simulink model "ASM_Traffic_V2X_Complete_Model_2"  (R2019a)
settings: Solver=ode1  StartTime=SIM.tstart.v  StopTime=Inf  FixedStep=SIM.StepSize.v  RelTol=1e-3
PostLoadFcn:
  | if any(exist('dsrtsu_mdlpostloadfcn', 'file') ~= 0), dsrtsu_mdlpostloadfcn('Execute', bdroot); end
  | try, asm_mdl_postloadfcn(bdroot, 'UpdateModel', 2200); catch, disp(lasterr); end,
undefined symbols (not defined in the file): _SensorPnts_1, _SensorPnts_13, _SensorPnts_17, _SensorPnts_21, _SensorPnts_25, _SensorPnts_29, _SensorPnts_33, _SensorPnts_37, _SensorPnts_41, _SensorPnts_45, _SensorPnts_49, _SensorPnts_5, _SensorPnts_53, _SensorPnts_57, _SensorPnts_9, _to_, CPT, G5A, ITS, MDL, rad, s_to_rpm, SIM
libraries: simulink x169, ASM_VehicleDynamics_lib x126, ASM_Traffic_lib x83, ASM_Utils_lib x49, mdbs x45, ASM_Environment_lib x17, dspindex x12, dsaV2xLibraryAux x10, dsmpblib x6, dsaV2xAsn1Library x4, dsaV2xLibrary x4, ASM_BrakeHydraulics_lib x4
(part 16 of 36)

== system ASM_Traffic_V2X_Complete_Model_2/MDLUserInterface/MotionDeskInterface/Fellow_VehicleLights/Fellow9 ==
  SW_Signals_UserInterface : Inport
  v_fellow[m|s] : Inport  Port=2
  TurnLights[0|1|2|3] : Inport  Port=3
  Acceleration[m|s2] : simulink/Discrete/Discrete Derivative  gainval=1.0  ICPrevScaledInput=0.0  OutMin=[]  OutMax=[]  OutDataType=fixdt(1, 16)  OutScaling=2^-10  DoSatur=off
  Bus Selector : BusSelector  OutputSignals=SW_ManualControl_Lights[1Scheduler|2Manual],SW_BrakeLight[0Off|1On],SW_TurnLights[0Off|1Left|2Right|3Both]
  Compare_Both : simulink/Logic and Bit Operations/Compare To Constant  relop===  const=3  OutDataTypeStr=boolean
  Compare_Brakelight : simulink/Logic and Bit Operations/Compare To Constant  relop=<  const=-0.2  OutDataTypeStr=boolean
  Compare_Turnlight_L : simulink/Logic and Bit Operations/Compare To Constant  relop===  const=1  OutDataTypeStr=boolean
  Compare_Turnlight_R : simulink/Logic and Bit Operations/Compare To Constant  relop===  const=2  OutDataTypeStr=boolean
  Data Type Conversion1 : DataTypeConversion  OutDataTypeStr=boolean
  Data Type Conversion2 : DataTypeConversion  OutDataTypeStr=uint32
  Data Type Conversion3 : DataTypeConversion  OutDataTypeStr=uint32
  Data Type Conversion4 : DataTypeConversion  OutDataTypeStr=uint32
  Logical Operator : Logic  Operator=OR  AllPortsSameDT=off  OutDataTypeStr=boolean
  Logical Operator1 : Logic  Operator=OR  AllPortsSameDT=off  OutDataTypeStr=boolean
  Multiport Switch : MultiPortSwitch  Inputs=2
  Multiport Switch4 : MultiPortSwitch  Inputs=2
  Mux16 : Mux  Inputs=3
  FellowLights : Outport
  wires:
  Data Type Conversion4/1 -> Multiport Switch4/2
  Data Type Conversion2/1 -> Multiport Switch4/3
  Data Type Conversion1/1 -> Multiport Switch/3
  Data Type Conversion3/1 -> Multiport Switch4/1, Multiport Switch/1
  SW_Signals_UserInterface/1 -> Bus Selector/1
  Acceleration[m|s2]/1 -> Compare_Brakelight/1
  Mux16/1 -> FellowLights/1
  TurnLights[0|1|2|3]/1 -> Data Type Conversion4/1
  v_fellow[m|s]/1 -> Acceleration[m|s2]/1
  Bus Selector/3 -> Data Type Conversion2/1  "<SW_TurnLights[0Off|1Left|2Right|3Both]>"
  Multiport Switch4/1 -> Compare_Both/1, Compare_Turnlight_R/1, Compare_Turnlight_L/1
  Logical Operator1/1 -> Mux16/3
  Logical Operator/1 -> Mux16/2
  Compare_Both/1 -> Logical Operator/2, Logical Operator1/2
  Compare_Turnlight_R/1 -> Logical Operator1/1
  Compare_Turnlight_L/1 -> Logical Operator/1
  Multiport Switch/1 -> Mux16/1
  Bus Selector/2 -> Data Type Conversion1/1  "<SW_BrakeLight[0Off|1On]>"
  Compare_Brakelight/1 -> Multiport Switch/2
  Bus Selector/1 -> Data Type Conversion3/1  "<SW_ManualControl_Lights[1Scheduler|2Manual]>"

== system ASM_Traffic_V2X_Complete_Model_2/MDLUserInterface/MotionDeskInterface/MOTION_DESK_INTERFACE/CalcLDWState ==
  NetworkItemType[] : Inport
  Dist_L[m] : Inport  Port=2
  Dist_R[m] : Inport  Port=3
  Compare To Constant : simulink/Logic and Bit Operations/Compare To Constant  relop===  const=3  OutDataTypeStr=boolean
  EvaluateDistance_L : If  IfExpression=u1 <= 0.01  ElseIfExpressions=(u1>0.01 & u1<=0.2)
  EvaluateDistance_R : If  IfExpression=u1 <= 0.01  ElseIfExpressions=(u1>0.01 & u1<=0.2)
  Junction : Constant  Value=0
  LeavingLane_L : Subsystem  TreatAsAtomicUnit=on
  LeavingLane_R : Subsystem  TreatAsAtomicUnit=on
  Merge : Merge  Inputs=3
  Merge1 : Merge  Inputs=3
  OK_L : Subsystem  TreatAsAtomicUnit=on
  OK_R : Subsystem  TreatAsAtomicUnit=on
  OutOfLane_L : Subsystem  TreatAsAtomicUnit=on
  OutOfLane_R : Subsystem  TreatAsAtomicUnit=on
  Switch : Switch  Criteria=u2 > Threshold
  Switch1 : Switch  Criteria=u2 > Threshold
  LDWState_L[] : Outport
  LDWState_R[] : Outport  Port=2
  wires:
  Merge1/1 -> Switch1/3
  Dist_R[m]/1 -> EvaluateDistance_R/1
  EvaluateDistance_R/1 -> OutOfLane_R/Action
  EvaluateDistance_R/2 -> LeavingLane_R/Action
  EvaluateDistance_R/3 -> OK_R/Action
  OutOfLane_R/1(Out1) -> Merge1/1
  LeavingLane_R/1(Out1) -> Merge1/2
  OK_R/1(Out1) -> Merge1/3
  Merge/1 -> Switch/3
  OK_L/1(Out1) -> Merge/3
  LeavingLane_L/1(Out1) -> Merge/2
  OutOfLane_L/1(Out1) -> Merge/1
  EvaluateDistance_L/3 -> OK_L/Action
  EvaluateDistance_L/2 -> LeavingLane_L/Action
  EvaluateDistance_L/1 -> OutOfLane_L/Action
  Dist_L[m]/1 -> EvaluateDistance_L/1
  Switch1/1 -> LDWState_R[]/1
  Junction/1 -> Switch/1, Switch1/1
  Switch/1 -> LDWState_L[]/1
  Compare To Constant/1 -> Switch/2, Switch1/2
  NetworkItemType[]/1 -> Compare To Constant/1

== system ASM_Traffic_V2X_Complete_Model_2/MDLUserInterface/MotionDeskInterface/MOTION_DESK_INTERFACE/Chassis ==
  Transform_In : Inport
  Pos_Vehicle_CoorSys_E[x;y;z][m] : Inport  Port=2
  Angle_Vehicle_CoorSys_E[x;y;z][deg] : Inport  Port=3
  MD_Object : mdbs/MD_Object  strObjId=0  strObjName=chassis  strBlockType=OBJ  bGUIEventOK=0
      settings: SourceProductName=dSPACE MotionDesk Blockset
  Selector : Selector  InputPortWidth=3  IndexOptions=Index vector (dialog)  Indices=[3 2 1]  OutputSizes=1
  Transform_Out : Outport
  wires:
  Selector/1 -> MD_Object/3
  Transform_In/1 -> MD_Object/1
  MD_Object/1 -> Transform_Out/1
  Pos_Vehicle_CoorSys_E[x;y;z][m]/1 -> MD_Object/2
  Angle_Vehicle_CoorSys_E[x;y;z][deg]/1 -> Selector/1

== system ASM_Traffic_V2X_Complete_Model_2/MDLUserInterface/MotionDeskInterface/MOTION_DESK_INTERFACE/Coding ==
  In1 : Inport
  Bitwise Operator3 : simulink/Logic and Bit Operations/Bitwise Operator  logicop=OR  UseBitMask=off  NumInputPorts=3  BitMask=bin2dec('11011001')  BitMaskRealWorld=Stored Integer
  Data Type Conversion : DataTypeConversion  OutDataTypeStr=uint32
  Data Type Conversion1 : DataTypeConversion  OutDataTypeStr=uint32
  Demux : Demux  Outputs=3
  Gain : Gain  Gain=15  ParamDataTypeStr=uint32  OutDataTypeStr=uint32
  Gain1 : Gain  Gain=15  ParamDataTypeStr=uint32  OutDataTypeStr=uint32
  Gain2 : Gain  Gain=15  ParamDataTypeStr=uint32  OutDataTypeStr=uint32
  Shift Arithmetic : ArithShift  BitShiftNumber=4  BitShiftDirection=Left
  Shift Arithmetic1 : ArithShift  BitShiftNumber=8  BitShiftDirection=Left
  SwitchDelay : Subsystem
  Out1 : Outport
  wires:
  Data Type Conversion1/1 -> Out1/1
  Bitwise Operator3/1 -> Data Type Conversion1/1
  Demux/1 -> Gain/1
  Data Type Conversion/1 -> Demux/1
  Shift Arithmetic1/1 -> Bitwise Operator3/3
  Shift Arithmetic/1 -> Bitwise Operator3/2
  Gain2/1 -> Shift Arithmetic1/1
  Gain1/1 -> Shift Arithmetic/1
  Gain/1 -> Bitwise Operator3/1
  In1/1 -> Data Type Conversion/1
  Demux/2 -> SwitchDelay/1(Turnlight_L)
  Demux/3 -> SwitchDelay/2(Turnlight_R)
  SwitchDelay/1(Turnlight_L_out) -> Gain1/1
  SwitchDelay/2(Turnlight_R_out) -> Gain2/1

== system ASM_Traffic_V2X_Complete_Model_2/MDLUserInterface/MotionDeskInterface/MOTION_DESK_INTERFACE/Coding_Fellows ==
  In1 : Inport
  Coding1 : Subsystem
  Coding10 : Subsystem
  Coding11 : Subsystem
  Coding12 : Subsystem
  Coding13 : Subsystem
  Coding14 : Subsystem
  Coding15 : Subsystem
  Coding2 : Subsystem
  Coding3 : Subsystem
  Coding4 : Subsystem
  Coding5 : Subsystem
  Coding6 : Subsystem
  Coding7 : Subsystem
  Coding8 : Subsystem
  Coding9 : Subsystem
  Demux : Demux  Outputs=15
  Mux : Mux  Inputs=15
  Out1 : Outport
  wires:
  In1/1 -> Demux/1
  Coding1/1(Out1) -> Mux/1
  Mux/1 -> Out1/1
  Coding2/1(Out1) -> Mux/2
  Coding3/1(Out1) -> Mux/3
  Coding4/1(Out1) -> Mux/4
  Coding5/1(Out1) -> Mux/5
  Coding6/1(Out1) -> Mux/6
  Coding7/1(Out1) -> Mux/7
  Coding8/1(Out1) -> Mux/8
  Coding9/1(Out1) -> Mux/9
  Coding10/1(Out1) -> Mux/10
  Coding11/1(Out1) -> Mux/11
  Coding12/1(Out1) -> Mux/12
  Coding13/1(Out1) -> Mux/13
  Coding14/1(Out1) -> Mux/14
  Coding15/1(Out1) -> Mux/15
  Demux/1 -> Coding1/1(In1)
  Demux/2 -> Coding2/1(In1)
  Demux/3 -> Coding3/1(In1)
  Demux/4 -> Coding4/1(In1)
  Demux/5 -> Coding5/1(In1)
  Demux/6 -> Coding6/1(In1)
  Demux/7 -> Coding7/1(In1)
  Demux/8 -> Coding8/1(In1)
  Demux/9 -> Coding9/1(In1)
  Demux/10 -> Coding10/1(In1)
  Demux/11 -> Coding11/1(In1)
  Demux/12 -> Coding12/1(In1)
  Demux/13 -> Coding13/1(In1)
  Demux/14 -> Coding14/1(In1)
  Demux/15 -> Coding15/1(In1)

== system ASM_Traffic_V2X_Complete_Model_2/MDLUserInterface/MotionDeskInterface/MOTION_DESK_INTERFACE/FrontAxle ==
  Transform_In : Inport
  Pos_Wheel_L[x;y;z][m] : Inport  Port=2
  AngleWheel_L[z;x][deg] : Inport  Port=3
  AngleWheel_L[y][deg] : Inport  Port=4
  r_Dyn_Tire_L[m] : Inport  Port=5
  F_Tire_L_CoorSys_V[x;y;z][N] : Inport  Port=6
  Pos_Wheel_R[x;y;z][m] : Inport  Port=7
  AngleWheel_R[z;x][deg] : Inport  Port=8
  AngleWheel_R[y][deg] : Inport  Port=9
  r_Dyn_Tire_R[m] : Inport  Port=10
  F_Tire_R_CoorSys_V[x;y;z][N] : Inport  Port=11
  Constant1 : Constant
  Constant2 : Constant  Value=0
  Constant8 : Constant  Value=0.36
  Demux2 : Demux  Outputs=3
  Demux4 : Demux  Outputs=3
  Divide : Product  Inputs=*/
  Divide1 : Product  Inputs=*/
  MD_Object1 : mdbs/MD_Object  strObjId=1  strObjName=wheel_FL  strBlockType=OBJ  bGUIEventOK=0
      settings: SourceProductName=dSPACE MotionDesk Blockset
  MD_Object2 : mdbs/MD_Object  strObjId=3  strObjName=_TireFrcs_F_LR  strBlockType=OBJ  bGUIEventOK=0
      settings: SourceProductName=dSPACE MotionDesk Blockset
  MD_Object5 : mdbs/MD_Object  strObjId=2  strObjName=wheel_FR  strBlockType=OBJ  bGUIEventOK=0
      settings: SourceProductName=dSPACE MotionDesk Blockset
  Mux{,1,4,8} (4 alike) : Mux  Inputs=3
  Mux2 : Mux  Inputs=8
  Mux3 : Mux  Inputs=2
  Mux5 : Mux  Inputs=2
  Pos_z_Offset_Arrow[m] : Constant  Value=0.1
  Product1 : Product  SaturateOnIntegerOverflow=on  OutDataTypeStr=Inherit: Same as first input
  Product2 : Product  SaturateOnIntegerOverflow=on  OutDataTypeStr=Inherit: Same as first input
  Reshape : Reshape  OutputDimensionality=Customize  OutputDimensions=[4,4]
  ScalingFaktor_F_Tire[] : Constant  Value=0.001
  Sign : Gain  Gain=-1
  Sum : Sum  Inputs=+-+  SaturateOnIntegerOverflow=on  InputSameDT=on  OutDataTypeStr=Inherit: Same as first input
  Sum1 : Sum  Inputs=+-+  SaturateOnIntegerOverflow=on  InputSameDT=on  OutDataTypeStr=Inherit: Same as first input
  Terminator1 : Terminator
  Terminator2 : Terminator
  Terminator5 : Terminator
  wires:
  AngleWheel_R[z;x][deg]/1 -> Mux5/1
  Sign/1 -> Mux3/1
  Mux5/1 -> MD_Object5/3
  Mux3/1 -> MD_Object1/3
  Reshape/1 -> MD_Object2/1
  Mux2/1 -> Reshape/1
  Constant2/1 -> Mux2/2, Mux2/4, Mux2/6, Mux2/8
  Product1/1 -> Mux2/7
  Mux1/1 -> Mux2/5
  Product2/1 -> Mux2/3
  Mux/1 -> Mux2/1
  AngleWheel_R[y][deg]/1 -> Mux5/2
  Transform_In/1 -> MD_Object1/1, MD_Object5/1
  r_Dyn_Tire_R[m]/1 -> Divide1/1, Sum1/2
  Constant1/1 -> Mux4/2, Mux8/2
  Mux8/1 -> MD_Object5/4
  Constant8/1 -> Divide/2, Divide1/2
  Divide1/1 -> Mux8/3, Mux8/1
  Pos_z_Offset_Arrow[m]/1 -> Sum1/3, Sum/3
  Sum1/1 -> Mux1/3
  Demux4/3 -> Sum1/1
  Demux4/2 -> Mux1/2
  Demux4/1 -> Mux1/1
  Pos_Wheel_R[x;y;z][m]/1 -> Demux4/1, MD_Object5/2
  ScalingFaktor_F_Tire[]/1 -> Product1/2, Product2/2
  F_Tire_R_CoorSys_V[x;y;z][N]/1 -> Product1/1
  MD_Object5/1 -> Terminator5/1
  MD_Object2/1 -> Terminator2/1
  MD_Object1/1 -> Terminator1/1
  F_Tire_L_CoorSys_V[x;y;z][N]/1 -> Product2/1
  Pos_Wheel_L[x;y;z][m]/1 -> MD_Object1/2, Demux2/1
  Demux2/1 -> Mux/1
  Demux2/2 -> Mux/2
  Demux2/3 -> Sum/1
  Sum/1 -> Mux/3
  Divide/1 -> Mux4/1, Mux4/3
  Mux4/1 -> MD_Object1/4
  r_Dyn_Tire_L[m]/1 -> Sum/2, Divide/1
  AngleWheel_L[z;x][deg]/1 -> Sign/1
  AngleWheel_L[y][deg]/1 -> Mux3/2

== system ASM_Traffic_V2X_Complete_Model_2/MDLUserInterface/MotionDeskInterface/MOTION_DESK_INTERFACE/LaneSensor1_L ==
  Transform_In : Inport
  Pos_Sensor[x;y;z][m] : Inport  Port=2
  Angle_Yaw[deg] : Inport  Port=3
  Scaling : Inport  Port=4
  Constant1 : Constant  Value=0
  Constant4 : Constant  Value=0
  MD_Object : mdbs/MD_Object  strObjId=38  strObjName=LaneSensor_Left  strBlockType=OBJ  bGUIEventOK=0
      settings: SourceProductName=dSPACE MotionDesk Blockset
  Mux : Mux  Inputs=3
  Mux1 : Mux  Inputs=3
  Terminator1 : Terminator
  wires:
  MD_Object/1 -> Terminator1/1
  Pos_Sensor[x;y;z][m]/1 -> MD_Object/2
  Transform_In/1 -> MD_Object/1
  Mux1/1 -> MD_Object/3
  Constant4/1 -> Mux1/3
  Constant1/1 -> Mux1/2
  Angle_Yaw[deg]/1 -> Mux1/1
  Mux/1 -> MD_Object/4
  Scaling/1 -> Mux/3, Mux/1, Mux/2

== system ASM_Traffic_V2X_Complete_Model_2/MDLUserInterface/MotionDeskInterface/MOTION_DESK_INTERFACE/LaneSensor1_R ==
  Transform_In : Inport
  Pos_Sensor[x;y;z][m] : Inport  Port=2
  Angle_Yaw[deg] : Inport  Port=3
  Scaling : Inport  Port=4
  Constant1 : Constant  Value=0
  Constant4 : Constant  Value=0
  MD_Object : mdbs/MD_Object  strObjId=39  strObjName=LaneSensor_Right  strBlockType=OBJ  bGUIEventOK=0
      settings: SourceProductName=dSPACE MotionDesk Blockset
  Mux : Mux  Inputs=3
  Mux1 : Mux  Inputs=3
  Terminator1 : Terminator
  wires:
  Constant4/1 -> Mux1/3
  Mux1/1 -> MD_Object/3
  Transform_In/1 -> MD_Object/1
  Pos_Sensor[x;y;z][m]/1 -> MD_Object/2
  MD_Object/1 -> Terminator1/1
  Constant1/1 -> Mux1/2
  Angle_Yaw[deg]/1 -> Mux1/1
  Scaling/1 -> Mux/3, Mux/1, Mux/2
  Mux/1 -> MD_Object/4

== system ASM_Traffic_V2X_Complete_Model_2/MDLUserInterface/MotionDeskInterface/MOTION_DESK_INTERFACE/RearAxle ==
  Transform_In : Inport
  Pos_Wheel_L[x;y;z][m] : Inport  Port=2
  AngleWheel_L[z;x][deg] : Inport  Port=3
  AngleWheel_L[y][deg] : Inport  Port=4
  r_Dyn_Tire_L[m] : Inport  Port=5
  F_Tire_L_CoorSys_V[x;y;z][N] : Inport  Port=6
  Pos_Wheel_R[x;y;z][m] : Inport  Port=7
  AngleWheel_R[z;x][deg] : Inport  Port=8
  AngleWheel_R[y][deg] : Inport  Port=9
  r_Dyn_Tire_R[m] : Inport  Port=10
  F_Tire_R_CoorSys_V[x;y;z][N] : Inport  Port=11
  Constant1 : Constant
  Constant2 : Constant  Value=0
  Constant8 : Constant  Value=0.36
  Demux2 : Demux  Outputs=3
  Demux4 : Demux  Outputs=3
  Divide : Product  Inputs=*/
  Divide1 : Product  Inputs=*/
  MD_Object1 : mdbs/MD_Object  strObjId=4  strObjName=wheel_RL  strBlockType=OBJ  bGUIEventOK=0
      settings: SourceProductName=dSPACE MotionDesk Blockset
  MD_Object5 : mdbs/MD_Object  strObjId=5  strObjName=wheel_RR  strBlockType=OBJ  bGUIEventOK=0
      settings: SourceProductName=dSPACE MotionDesk Blockset
  MD_Object6 : mdbs/MD_Object  strObjId=6  strObjName=_TireFrcs_R_LR  strBlockType=OBJ  bGUIEventOK=0
      settings: SourceProductName=dSPACE MotionDesk Blockset
  Mux{,1,4,8} (4 alike) : Mux  Inputs=3
  Mux2 : Mux  Inputs=8
  Mux3 : Mux  Inputs=2
  Mux5 : Mux  Inputs=2
  Pos_z_Offset_Arrow[m] : Constant  Value=0.1
  Product1 : Product  SaturateOnIntegerOverflow=on  OutDataTypeStr=Inherit: Same as first input
  Product2 : Product  SaturateOnIntegerOverflow=on  OutDataTypeStr=Inherit: Same as first input
  Reshape : Reshape  OutputDimensionality=Customize  OutputDimensions=[4,4]
  ScalingFaktor_F_Tire[] : Constant  Value=0.001
  Sign : Gain  Gain=-1
  Sum : Sum  Inputs=+-+  SaturateOnIntegerOverflow=on  InputSameDT=on  OutDataTypeStr=Inherit: Same as first input
  Sum1 : Sum  Inputs=+-+  SaturateOnIntegerOverflow=on  InputSameDT=on  OutDataTypeStr=Inherit: Same as first input
  Terminator1 : Terminator
  Terminator5 : Terminator
  Terminator6 : Terminator
  wires:
  Sign/1 -> Mux3/1
  Mux5/1 -> MD_Object5/3
  Mux3/1 -> MD_Object1/3
  Product1/1 -> Mux2/7
  Mux1/1 -> Mux2/5
  Product2/1 -> Mux2/3
  Mux/1 -> Mux2/1
  Reshape/1 -> MD_Object6/1
  Mux2/1 -> Reshape/1
  Constant2/1 -> Mux2/2, Mux2/4, Mux2/6, Mux2/8
  MD_Object5/1 -> Terminator5/1
  MD_Object6/1 -> Terminator6/1
  F_Tire_R_CoorSys_V[x;y;z][N]/1 -> Product1/1
  ScalingFaktor_F_Tire[]/1 -> Product2/2, Product1/2
  Pos_Wheel_R[x;y;z][m]/1 -> MD_Object5/2, Demux4/1
  Demux4/1 -> Mux1/1
  Demux4/2 -> Mux1/2
  Demux4/3 -> Sum1/1
  Sum1/1 -> Mux1/3
  Pos_z_Offset_Arrow[m]/1 -> Sum/3, Sum1/3
  Divide1/1 -> Mux8/1, Mux8/3
  Constant8/1 -> Divide/2, Divide1/2
  Mux8/1 -> MD_Object5/4
  Constant1/1 -> Mux4/2, Mux8/2
  r_Dyn_Tire_R[m]/1 -> Sum1/2, Divide1/1
  Transform_In/1 -> MD_Object1/1, MD_Object5/1
  AngleWheel_R[z;x][deg]/1 -> Mux5/1
  AngleWheel_R[y][deg]/1 -> Mux5/2
  MD_Object1/1 -> Terminator1/1
  F_Tire_L_CoorSys_V[x;y;z][N]/1 -> Product2/1
  Pos_Wheel_L[x;y;z][m]/1 -> Demux2/1, MD_Object1/2
  Demux2/1 -> Mux/1
  Demux2/2 -> Mux/2
  Demux2/3 -> Sum/1
  Sum/1 -> Mux/3
  Divide/1 -> Mux4/1, Mux4/3
  Mux4/1 -> MD_Object1/4
  r_Dyn_Tire_L[m]/1 -> Sum/2, Divide/1
  AngleWheel_L[z;x][deg]/1 -> Sign/1
  AngleWheel_L[y][deg]/1 -> Mux3/2

== system ASM_Traffic_V2X_Complete_Model_2/MDLUserInterface/MotionDeskInterface/MOTION_DESK_INTERFACE/SteeringWheel ==
  Transform_In : Inport
  Angle_SteeringWheel[deg] : Inport  Port=2
  Angle_inclination[deg] : Constant  Value=205
  MD_Object3 : mdbs/MD_Object  strObjId=7  strObjName=steering_wheel  strBlockType=OBJ  bGUIEventOK=0
      settings: SourceProductName=dSPACE MotionDesk Blockset
  Mux : Mux  Inputs=3
  Pos_SteeringWheel[m] : Constant  Value=[-1.3, 0.35, 0.53]
  Terminator3 : Terminator
  const : Constant  Value=0
  wires:
  Angle_SteeringWheel[deg]/1 -> Mux/3
  Pos_SteeringWheel[m]/1 -> MD_Object3/2
  Mux/1 -> MD_Object3/3
  Transform_In/1 -> MD_Object3/1
  Angle_inclination[deg]/1 -> Mux/2
  const/1 -> Mux/1
  MD_Object3/1 -> Terminator3/1

== system ASM_Traffic_V2X_Complete_Model_2/MDLUserInterface/MotionDeskInterface/MOTION_DESK_INTERFACE/Traffic_Animation ==
  Transform_In : Inport
  Pos_Fellows_MainPnt_CoorSys_E[x;y;z][m] : Inport  Port=2
  Angle_Fellows[x;y;z][deg] : Inport  Port=3
  Flag_FellowsUsed[0|1] : Inport  Port=4
  Sensors_Signals : Inport  Port=5
  Fellows_Animation : Subsystem
  Sensors_Animation : Subsystem
  wires:
  Transform_In/1 -> Sensors_Animation/1(Transform_In)
  Sensors_Signals/1 -> Sensors_Animation/2(Sensors_Signals)
  Flag_FellowsUsed[0|1]/1 -> Fellows_Animation/3(Flag_FellowsUsed[0|1])
  Pos_Fellows_MainPnt_CoorSys_E[x;y;z][m]/1 -> Fellows_Animation/1(Pos_Fellows_MainPnt_CoorSys_E[x;y;z][m])
  Angle_Fellows[x;y;z][deg]/1 -> Fellows_Animation/2(Angle_Fellows[x;y;z][deg])

== system ASM_Traffic_V2X_Complete_Model_2/MDLUserInterface/SoftECU/MDL_DISP/SoftECU_ACC ==
  ASMSignalBus_ACC : Inport
  ASMSignalBus_Vehicle : Inport  Port=2
  ACC_Control_Mode[0OFF|1CC|2DC] : Subsystem
      mask Display: disp('')
  ACC_State[0OFF|2Standby|3ON] : Subsystem
      mask Display: disp('')
  AEB[0Off|1On] : Subsystem
      mask Display: disp('')
  Bus Selector1 : BusSelector  OutputSignals=Controller_ACC.State_ACC[0Off|1On],Controller_ACC.Control_Mode_ACC[0Off|1CC|2DC],Controller_ACC.FCW[0Off|1On],Controller_ACC.AEB[0Off|1On],Controller_ACC.TTC[s],Controller_ACC.Collision[0Off|1On],Controller_ACC.Sw_BrakeMode[1Comfort|2AEBOnly|3AEBOff]
  Bus Selector3 : BusSelector  OutputSignals=Controller_ACC.Control_Mode_ACC[0Off|1CC|2DC],Controller_ACC.v_Set[km|h],Target_Selection_ACC.v_Rel[m|s],Controller_ACC.Distance_Set[m],Target_Selection_ACC.Dist_Long[m],Interface_ACC.Trq_Request_Brake_ACC[Nm],Interface_ACC.Trq_Request_Engine_ACC[Nm],Operator_Interface_ACC.ACC_State[1OFF|2Standby|3ON],Target_Selection_ACC.Target_Detected[0|1]
  Bus Selector5 : BusSelector  OutputSignals=VehicleMovement.Velocities.Vehicle.Linear.v_Total_Vehicle[km|h]
  Collision[0Off|1On] : Subsystem
      mask Display: disp('')
  Control_Mode_ACC[0Off|1CC|2DC] : Subsystem
      mask Display: disp('')
  Dist_Long[m] : Subsystem
      mask Display: disp('')
  Distance_Set[m] : Subsystem
      mask Display: disp('')
  FCW[0Off|1On] : Subsystem
      mask Display: disp('')
  Mux1 : Mux  Inputs=2
  Mux3 : Mux  Inputs=2
  SoftECU_ACC : Scope  NumInputPorts=6
  SoftECU_ACC_States : Scope  NumInputPorts=7
  State_ACC[0Off|1On] : Subsystem
      mask Display: disp('')
  Sw_BrakeMode[1Comfort|2AEBOnly|3AEBOff] : Subsystem
      mask Display: disp('')
  TTC[s] : Subsystem
      mask Display: disp('')
  Target_Detected[0|1] : Subsystem
      mask Display: disp('')
  Terminator : Terminator
  Terminator1 : Terminator
  Trq_Request_Brake_ACC[Nm] : Subsystem
      mask Display: disp('')
  Trq_Request_Engine_ACC[Nm] : Subsystem
      mask Display: disp('')
  UnitConversion : ASM_Utils_lib/UnitConversion/UnitConversion  Selection=m/s_to_km/h
  v_Rel[km|h] : Subsystem
      mask Display: disp('')
  v_Set[km|h] : Subsystem
      mask Display: disp('')
  wires:
  ASMSignalBus_ACC/1 -> Bus Selector1/1, Bus Selector3/1
  ASMSignalBus_Vehicle/1 -> Bus Selector5/1
  Bus Selector1/5 -> TTC[s]/1(In1)  "<TTC[s]>"
  Bus Selector1/3 -> FCW[0Off|1On]/1(In1)  "<FCW[0Off|1On]>"
  Bus Selector1/4 -> AEB[0Off|1On]/1(In1)  "<AEB[0Off|1On]>"
  Bus Selector1/1 -> State_ACC[0Off|1On]/1(In1)  "<State_ACC[0Off|1On]>"
  Bus Selector1/2 -> Control_Mode_ACC[0Off|1CC|2DC]/1(In1)  "<Control_Mode_ACC[0Off|1CC|2DC]>"
  Bus Selector1/6 -> Collision[0Off|1On]/1(In1)  "<Collision[0Off|1On]>"
  Bus Selector1/7 -> Sw_BrakeMode[1Comfort|2AEBOnly|3AEBOff]/1(In1)  "<Sw_BrakeMode[1Comfort|2AEBOnly|3AEBOff]>"
  State_ACC[0Off|1On]/1(Out1) -> SoftECU_ACC_States/1  "State_ACC[0Off|1On]"
  Control_Mode_ACC[0Off|1CC|2DC]/1(Out1) -> SoftECU_ACC_States/2  "Control_Mode_ACC[0Off|1CC|2DC]"
  FCW[0Off|1On]/1(Out1) -> SoftECU_ACC_States/3  "FCW[0Off|1On]"
  AEB[0Off|1On]/1(Out1) -> SoftECU_ACC_States/4  "AEB[0Off|1On]"
  TTC[s]/1(Out1) -> SoftECU_ACC_States/5  "TTC[s]"
  Collision[0Off|1On]/1(Out1) -> SoftECU_ACC_States/6  "Collision[0Off|1On]"
  Sw_BrakeMode[1Comfort|2AEBOnly|3AEBOff]/1(Out1) -> SoftECU_ACC_States/7  "Sw_BrakeMode[1Comfort|2AEBOnly|3AEBOff]"
  Bus Selector3/1 -> ACC_Control_Mode[0OFF|1CC|2DC]/1(In1)  "<Control_Mode_ACC[0Off|1CC|2DC]>"
  Bus Selector3/2 -> v_Set[km|h]/1(In1)  "<v_Set[km|h]>"
  Bus Selector3/3 -> UnitConversion/1  "<v_Rel[m|s]>"
  Bus Selector3/4 -> Distance_Set[m]/1(In1)  "<Distance_Set[m]>"
  Bus Selector3/5 -> Dist_Long[m]/1(In1)  "<Dist_Long[m]>"
  Bus Selector3/6 -> Trq_Request_Brake_ACC[Nm]/1(In1)  "<Trq_Request_Brake_ACC[Nm]>"
  Bus Selector3/7 -> Trq_Request_Engine_ACC[Nm]/1(In1)  "<Trq_Request_Engine_ACC[Nm]>"
  v_Set[km|h]/1(Out1) -> Mux3/1
  Distance_Set[m]/1(Out1) -> Mux1/1
  Dist_Long[m]/1(Out1) -> Mux1/2
  Bus Selector5/1 -> Mux3/2  "<v_Total_Vehicle[km|h]>"
  ACC_Control_Mode[0OFF|1CC|2DC]/1(Out1) -> SoftECU_ACC/1  "ACC_Control_Mode[0OFF|1CC|2DC]"
  Mux3/1 -> SoftECU_ACC/2  "Velocity[km|h]"
  UnitConversion/1 -> v_Rel[km|h]/1(In1)
  v_Rel[km|h]/1(Out1) -> SoftECU_ACC/3  "v_Rel[km|h]"
  Mux1/1 -> SoftECU_ACC/4  "Distance[m]"
  Trq_Request_Brake_ACC[Nm]/1(Out1) -> SoftECU_ACC/5  "Trq_Request_Brake_ACC[Nm]"
  Trq_Request_Engine_ACC[Nm]/1(Out1) -> SoftECU_ACC/6  "Trq_Request_Engine_ACC[Nm]"
  Bus Selector3/8 -> ACC_State[0OFF|2Standby|3ON]/1(In1)  "<ACC_State[1OFF|2Standby|3ON]>"
  Bus Selector3/9 -> Target_Detected[0|1]/1(In1)  "<Target_Detected[0|1]>"
  ACC_State[0OFF|2Standby|3ON]/1(Out1) -> Terminator/1
  Target_Detected[0|1]/1(Out1) -> Terminator1/1

== system ASM_Traffic_V2X_Complete_Model_2/MDLUserInterface/SoftECU/MDL_DISP/SoftECU_Body ==
  In : Inport
  Bus Selector3 : BusSelector  OutputSignals=Flag_NotPressed_Pedal[0|1],Sw_Ignition[0|1],Sw_StarterReq[0|1],State_StartButton[-2|-1|0|1|2|3]
  Flag_NotPressed_Pedal[0|1] : Subsystem
      mask Display: disp('')
  START_BUTTON : Scope  NumInputPorts=4
  StartStateButtonLogic : Subsystem
  State_StartButton[-2NotAuthorized|-1PowerOff|0Acc|1PowerOn|2StarterOn|3EngRunning] : Subsystem
      mask Display: disp('')
  Sw_Ignition[0|1] : Subsystem
      mask Display: disp('')
  Sw_StarterReq[0|1] : Subsystem
      mask Display: disp('')
  wires:
  Bus Selector3/4 -> StartStateButtonLogic/1(In1)  "<State_StartButton[-2|-1|0|1|2|3]>"
  State_StartButton[-2NotAuthorized|-1PowerOff|0Acc|1PowerOn|2StarterOn|3EngRunning]/1(Out1) -> START_BUTTON/4  "State_StartButton[-2NotAuthorized|-1PowerOff|0Acc|1PowerOn|2StarterOn|3EngRunning]"
  Bus Selector3/3 -> Sw_StarterReq[0|1]/1(In1)  "<Sw_StarterReq[0|1]>"
  Bus Selector3/2 -> Sw_Ignition[0|1]/1(In1)  "<Sw_Ignition[0|1]>"
  Bus Selector3/1 -> Flag_NotPressed_Pedal[0|1]/1(In1)  "<Flag_NotPressed_Pedal[0|1]>"
  Sw_Ignition[0|1]/1(Out1) -> START_BUTTON/2  "Sw_Ignition[0|1]"
  Sw_StarterReq[0|1]/1(Out1) -> START_BUTTON/3  "Sw_StarterReq[0|1]"
  Flag_NotPressed_Pedal[0|1]/1(Out1) -> START_BUTTON/1  "Flag_NotPressed_Pedal[0|1]"
  In/1 -> Bus Selector3/1
  StartStateButtonLogic/1(Out1) -> State_StartButton[-2NotAuthorized|-1PowerOff|0Acc|1PowerOn|2StarterOn|3EngRunning]/1(In1)

== system ASM_Traffic_V2X_Complete_Model_2/MDLUserInterface/SoftECU/MDL_DISP/SoftECU_Brake ==
  ASMSignalBus : Inport
  Bus Selector1 : BusSelector  OutputSignals=DesiredBrakePressure.Enable_p_Brake_Desired[0|1],DesiredBrakePressure.p_Brake_Desired[bar]
  Enable_p_Brake_Desired[0|1] : Subsystem
      mask Display: disp('')
  SoftECU_Brake : Scope  NumInputPorts=2
  p_Brake_Desired[bar] : Subsystem
      mask Display: disp('')
  wires:
  p_Brake_Desired[bar]/1(Out1) -> SoftECU_Brake/2  "p_Brake_Desired[bar]"
  Enable_p_Brake_Desired[0|1]/1(Out1) -> SoftECU_Brake/1  "Enable_p_Brake_Desired[0|1]"
  ASMSignalBus/1 -> Bus Selector1/1
  Bus Selector1/2 -> p_Brake_Desired[bar]/1(In1)  "<p_Brake_Desired[bar]>"
  Bus Selector1/1 -> Enable_p_Brake_Desired[0|1]/1(In1)  "<Enable_p_Brake_Desired[0|1]>"

== system ASM_Traffic_V2X_Complete_Model_2/MDLUserInterface/SoftECU/MDL_DISP/SoftECU_Engine ==
  ASMSignalBus : Inport
  Bus Selector1 : BusSelector  OutputSignals=TorqueIntervention_Fast.Enable_Trq_Intervention_Fast[0|1],TorqueIntervention_Fast.Trq_Request_Fast[Nm],TorqueIntervention_Slow.Enable_TrqDecrease_ESP[0|1],TorqueIntervention_Slow.Trq_DecreaseRequest_ESP[Nm],TorqueIntervention_Slow.Pos_AccPedal_Request_Fast_ESP[%],TorqueIntervention_Slow.Pos_AccPedal_Request_Slow_ESP[%],TorqueIntervention_Slow.Enable_TrqDecrease_Extern[0|1],TorqueIntervention_Slow.Pos_AccPedal_Request_Extern[%],IdleSpeedControl.Pos_AccPedal[%],TorqueIntervention_Slow.Pos_AccPedal_Influenced[%]
  Enable_TrqDecrease_ESP[0|1] : Subsystem
      mask Display: disp('')
  Enable_TrqDecrease_Extern[0|1] : Subsystem
      mask Display: disp('')
  Enable_Trq_Intervention_Fast[0|1] : Subsystem
      mask Display: disp('')
  Mux : Mux  Inputs=2
  Mux1 : Mux  Inputs=2
  Pos_AccPedal[%] : Subsystem
      mask Display: disp('')
  Pos_AccPedal_Influenced[%] : Subsystem
      mask Display: disp('')
  Pos_AccPedal_Request_Extern[%] : Subsystem
      mask Display: disp('')
  Pos_AccPedal_Request_Fast_ESP[%] : Subsystem
      mask Display: disp('')
  Pos_AccPedal_Request_Slow_ESP[%]1 : Subsystem
      mask Display: disp('')
  SoftECU_Engine_TorqueIntervention_Fast : Scope  NumInputPorts=2
  SoftECU_Engine_TorqueIntervention_Slow : Scope  NumInputPorts=6
  Trq_DecreaseRequest_ESP[Nm] : Subsystem
      mask Display: disp('')
  Trq_Request_Fast[Nm] : Subsystem
      mask Display: disp('')
  wires:
  Bus Selector1/10 -> Pos_AccPedal_Influenced[%]/1(In1)  "<Pos_AccPedal_Influenced[%]>"
  Bus Selector1/9 -> Pos_AccPedal[%]/1(In1)  "<Pos_AccPedal[%]>"
  Bus Selector1/8 -> Pos_AccPedal_Request_Extern[%]/1(In1)  "<Pos_AccPedal_Request_Extern[%]>"
  Bus Selector1/7 -> Enable_TrqDecrease_Extern[0|1]/1(In1)  "<Enable_TrqDecrease_Extern[0|1]>"
  Bus Selector1/6 -> Pos_AccPedal_Request_Slow_ESP[%]1/1(In1)  "<Pos_AccPedal_Request_Slow_ESP[%]>"
  Mux1/1 -> SoftECU_Engine_TorqueIntervention_Slow/3  "Pos_AccPedal_Request_ESP[%]"
  Pos_AccPedal_Request_Slow_ESP[%]1/1(Out1) -> Mux1/2
  Pos_AccPedal_Request_Fast_ESP[%]/1(Out1) -> Mux1/1
  Mux/1 -> SoftECU_Engine_TorqueIntervention_Slow/6  "Pos_AccPedal[%]"
  Pos_AccPedal_Request_Extern[%]/1(Out1) -> SoftECU_Engine_TorqueIntervention_Slow/5  "Pos_AccPedal_Request_Extern[%]"
  Enable_TrqDecrease_Extern[0|1]/1(Out1) -> SoftECU_Engine_TorqueIntervention_Slow/4  "Enable_TrqDecrease_Extern[0|1]"
  Trq_DecreaseRequest_ESP[Nm]/1(Out1) -> SoftECU_Engine_TorqueIntervention_Slow/2  "Trq_DecreaseRequest_ESP[Nm]"
  Enable_TrqDecrease_ESP[0|1]/1(Out1) -> SoftECU_Engine_TorqueIntervention_Slow/1  "Enable_TrqDecrease_ESP[0|1]"
  Pos_AccPedal_Influenced[%]/1(Out1) -> Mux/2
  Pos_AccPedal[%]/1(Out1) -> Mux/1
  Trq_Request_Fast[Nm]/1(Out1) -> SoftECU_Engine_TorqueIntervention_Fast/2  "Trq_Request_Fast[Nm]"
  Enable_Trq_Intervention_Fast[0|1]/1(Out1) -> SoftECU_Engine_TorqueIntervention_Fast/1  "Enable_Trq_Intervention_Fast[0|1]"
  ASMSignalBus/1 -> Bus Selector1/1
  Bus Selector1/5 -> Pos_AccPedal_Request_Fast_ESP[%]/1(In1)  "<Pos_AccPedal_Request_Fast_ESP[%]>"
  Bus Selector1/4 -> Trq_DecreaseRequest_ESP[Nm]/1(In1)  "<Trq_DecreaseRequest_ESP[Nm]>"
  Bus Selector1/3 -> Enable_TrqDecrease_ESP[0|1]/1(In1)  "<Enable_TrqDecrease_ESP[0|1]>"
  Bus Selector1/2 -> Trq_Request_Fast[Nm]/1(In1)  "<Trq_Request_Fast[Nm]>"
  Bus Selector1/1 -> Enable_Trq_Intervention_Fast[0|1]/1(In1)  "<Enable_Trq_Intervention_Fast[0|1]>"

== system ASM_Traffic_V2X_Complete_Model_2/MDLUserInterface/SoftECU/MDL_DISP/SoftECU_Transmission ==
  ASMSignalBus : Inport
  Bus Selector1 : BusSelector  OutputSignals=Lockup_Clutch_Control.Ctrl_Lockup_Clutch[%],Torque_Intervention_Control.Gear[],Torque_Intervention_Control.Factor_Trq_Engine_Red[%],Shift_Lock_Control.Ctrl_Parking_Pawl[0|1]
  Ctrl_Lockup_Clutch[%] : Subsystem
      mask Display: disp('')
  Ctrl_Parking_Pawl[0|1] : Subsystem
      mask Display: disp('')
  Factor_Trq_Engine_Red[%] : Subsystem
      mask Display: disp('')
  Gear[] : Subsystem
      mask Display: disp('')
  SoftECU_Transmission : Scope  NumInputPorts=4
  wires:
  Bus Selector1/1 -> Ctrl_Lockup_Clutch[%]/1(In1)  "<Ctrl_Lockup_Clutch[%]>"
  Ctrl_Lockup_Clutch[%]/1(Out1) -> SoftECU_Transmission/1  "Ctrl_Lockup_Clutch[%]"
  Bus Selector1/2 -> Gear[]/1(In1)  "<Gear[]>"
  Gear[]/1(Out1) -> SoftECU_Transmission/2  "Gear[]"
  Bus Selector1/4 -> Ctrl_Parking_Pawl[0|1]/1(In1)  "<Ctrl_Parking_Pawl[0|1]>"
  Ctrl_Parking_Pawl[0|1]/1(Out1) -> SoftECU_Transmission/4  "Ctrl_Parking_Pawl[0|1]"
  ASMSignalBus/1 -> Bus Selector1/1
  Bus Selector1/3 -> Factor_Trq_Engine_Red[%]/1(In1)  "<Factor_Trq_Engine_Red[%]>"
  Factor_Trq_Engine_Red[%]/1(Out1) -> SoftECU_Transmission/3  "Factor_Trq_Engine_Red[%]"

== system ASM_Traffic_V2X_Complete_Model_2/MDLUserInterface/SoftECU/MDL_PAR/SoftECU_ESP_Switches ==
  Bus Creator : BusCreator  Inputs=3
  SW_ASR[0Off|1On] : Constant
  Sw_ESP[0Off|1ABS|2ESP] : Constant  Value=2
  Sw_ESP_Control_Mode[1ManSched|2Manual] : Constant
  tag scope: TAG_SoftECU_ESP_Switches=global
  wires:
  Sw_ESP_Control_Mode[1ManSched|2Manual]/1 -> Bus Creator/1  "Sw_ESP_Control_Mode[1ManSched|2Manual]"
  SW_ASR[0Off|1On]/1 -> Bus Creator/3  "SW_ASR[0Off|1On]"
  Bus Creator/1 -> [TAG_SoftECU_ESP_Switches]
  Sw_ESP[0Off|1ABS|2ESP]/1 -> Bus Creator/2  "Sw_ESP[0Off|1ABS|2ESP]"

== system ASM_Traffic_V2X_Complete_Model_2/MDLUserInterface/SoftECU/MDL_PAR/SoftECU_StartButton_Switches ==
  State_KeyFob[1NotAuthorized|2Authorized] : Constant  Value=2
  tag scope: TAG_SoftECU_State_KeyFob=global
  wires:
  State_KeyFob[1NotAuthorized|2Authorized]/1 -> [TAG_SoftECU_State_KeyFob]

== system ASM_Traffic_V2X_Complete_Model_2/MDLUserInterface/VehicleDynamics/MDL_DISP/Accelerations ==
  Accelerations : Inport
  AngularAccelerations : Scope
  Bus Selector2 : BusSelector  OutputSignals=VehicleCoG.Linear.a_Vehicle_CoG[x;y;z][m|s2].a_x_Vehicle_CoG[m|s2],VehicleCoG.Linear.a_Vehicle_CoG[x;y;z][m|s2].a_y_Vehicle_CoG[m|s2],VehicleCoG.Linear.a_Vehicle_CoG[x;y;z][m|s2].a_z_Vehicle_CoG[m|s2],VehicleCoG.Angular.w_Vehicle_CoG_dt[x;y;z][rad|s2],VehicleCoG.Angular.w_Vehicle_CoG_dt[x;y;z][rad|s2].w_x_Vehicle_CoG_dt[rad|s2],VehicleCoG.Angular.w_Vehicle_CoG_dt[x;y;z][rad|s2].w_y_Vehicle_CoG_dt[rad|s2],VehicleCoG.Angular.w_Vehicle_CoG_dt[x;y;z][rad|s2].w_z_Vehicle_CoG_dt[rad|s2],Wheels.Linear.a_FL_Wheel[x;y;z][m|s2],Wheels.Linear.a_FR_Wheel[x;y;z][m|s2],Wheels.Linear.a_RL_Wheel[x;y;z][m|s2],Wheels.Linear.a_RR_Wheel[x;y;z][m|s2]
  Mux : Mux  Inputs=3
  Terminator : Terminator
  TransAccelerations : Scope  NumInputPorts=3
  WheelLinearAccelerations : Scope  NumInputPorts=4
  a_FL_Wheel[x;y;z][m|s2] : Subsystem
      mask Display: disp('')
  a_FR_Wheel[x;y;z][m|s2] : Subsystem
      mask Display: disp('')
  a_RL_Wheel[x;y;z][m|s2] : Subsystem
      mask Display: disp('')
  a_RR_Wheel[x;y;z][m|s2] : Subsystem
      mask Display: disp('')
  a_x_Vehicle_CoG[m|s2] : Subsystem
      mask Display: disp('')
  a_y_Vehicle_CoG[m|s2] : Subsystem
      mask Display: disp('')
  a_z_Vehicle_CoG[m|s2] : Subsystem
      mask Display: disp('')
  w_Vehicle_CoG_dt[x;y;z][rad|s2] : Subsystem
      mask Display: disp('')
  w_x_Vehicle_CoG_dt[rad|s2] : Subsystem
      mask Display: disp('')
  w_y_Vehicle_CoG_dt[rad|s2] : Subsystem
      mask Display: disp('')
  w_z_Vehicle_CoG_dt[rad|s2] : Subsystem
      mask Display: disp('')
  wires:
  Mux/1 -> AngularAccelerations/1  "w_Vehicle_CoG_dt[x;y;z][rad|s2]"
  w_z_Vehicle_CoG_dt[rad|s2]/1(Out1) -> Mux/3
  w_y_Vehicle_CoG_dt[rad|s2]/1(Out1) -> Mux/2
  w_x_Vehicle_CoG_dt[rad|s2]/1(Out1) -> Mux/1
  Bus Selector2/7 -> w_z_Vehicle_CoG_dt[rad|s2]/1(In1)  "<w_z_Vehicle_CoG_dt[rad|s2]>"
  Bus Selector2/6 -> w_y_Vehicle_CoG_dt[rad|s2]/1(In1)  "<w_y_Vehicle_CoG_dt[rad|s2]>"
  Bus Selector2/5 -> w_x_Vehicle_CoG_dt[rad|s2]/1(In1)  "<w_x_Vehicle_CoG_dt[rad|s2]>"
  Bus Selector2/3 -> a_z_Vehicle_CoG[m|s2]/1(In1)  "<a_z_Vehicle_CoG[m|s2]>"
  Bus Selector2/2 -> a_y_Vehicle_CoG[m|s2]/1(In1)  "<a_y_Vehicle_CoG[m|s2]>"
  Bus Selector2/1 -> a_x_Vehicle_CoG[m|s2]/1(In1)  "<a_x_Vehicle_CoG[m|s2]>"
  Bus Selector2/11 -> a_RR_Wheel[x;y;z][m|s2]/1(In1)  "<a_RR_Wheel[x;y;z][m|s2]>"
  Bus Selector2/10 -> a_RL_Wheel[x;y;z][m|s2]/1(In1)  "<a_RL_Wheel[x;y;z][m|s2]>"
  Bus Selector2/9 -> a_FR_Wheel[x;y;z][m|s2]/1(In1)  "<a_FR_Wheel[x;y;z][m|s2]>"
  Bus Selector2/8 -> a_FL_Wheel[x;y;z][m|s2]/1(In1)  "<a_FL_Wheel[x;y;z][m|s2]>"
  a_RR_Wheel[x;y;z][m|s2]/1(Out1) -> WheelLinearAccelerations/4  "a_RR_Wheel[x;y;z][m|s2]"
  a_RL_Wheel[x;y;z][m|s2]/1(Out1) -> WheelLinearAccelerations/3  "a_RL_Wheel[x;y;z][m|s2]"
  a_FR_Wheel[x;y;z][m|s2]/1(Out1) -> WheelLinearAccelerations/2  "a_FR_Wheel[x;y;z][m|s2]"
  a_FL_Wheel[x;y;z][m|s2]/1(Out1) -> WheelLinearAccelerations/1  "a_FL_Wheel[x;y;z][m|s2]"
  a_z_Vehicle_CoG[m|s2]/1(Out1) -> TransAccelerations/3  "a_z_Vehicle_CoG[m|s2]"
  a_y_Vehicle_CoG[m|s2]/1(Out1) -> TransAccelerations/2  "a_y_Vehicle_CoG[m|s2]"
  a_x_Vehicle_CoG[m|s2]/1(Out1) -> TransAccelerations/1  "a_x_Vehicle_CoG[m|s2]"
  Accelerations/1 -> Bus Selector2/1
  Bus Selector2/4 -> w_Vehicle_CoG_dt[x;y;z][rad|s2]/1(In1)  "<w_Vehicle_CoG_dt[x;y;z][rad|s2]>"
  w_Vehicle_CoG_dt[x;y;z][rad|s2]/1(Out1) -> Terminator/1  "w_Vehicle_CoG_dt[x;y;z][rad|s2]"

== system ASM_Traffic_V2X_Complete_Model_2/MDLUserInterface/VehicleDynamics/MDL_DISP/Aerodynamics ==
  Aerodynamics : Inport
  Aerodynamics1 : Scope  NumInputPorts=2
  Bus Selector5 : BusSelector  OutputSignals=Forces.F_x_Aero_CoorSys_V[N],Forces.F_y_Aero_CoorSys_V[N],Forces.F_z_Aero_CoorSys_V[N],Torques.Trq_x_Aero_CoorSys_V[Nm],Torques.Trq_y_Aero_CoorSys_V[Nm],Torques.Trq_z_Aero_CoorSys_V[Nm]
  F_x_Aero_CoorSys_V[N] : Subsystem
      mask Display: disp('')
  F_y_Aero_CoorSys_V[N] : Subsystem
      mask Display: disp('')
  F_z_Aero_CoorSys_V[N] : Subsystem
      mask Display: disp('')
  Mux : Mux  Inputs=3
  Mux1 : Mux  Inputs=3
  Trq_x_Aero_CoorSys_V[Nm] : Subsystem
      mask Display: disp('')
  Trq_y_Aero_CoorSys_V[Nm] : Subsystem
      mask Display: disp('')
  Trq_z_Aero_CoorSys_V[Nm] : Subsystem
      mask Display: disp('')
  wires:
  Trq_z_Aero_CoorSys_V[Nm]/1(Out1) -> Mux1/3  "Trq_z_Aero_CoorSys_V[Nm]"
  Bus Selector5/6 -> Trq_z_Aero_CoorSys_V[Nm]/1(In1)  "<Trq_z_Aero_CoorSys_V[Nm]>"
  Trq_y_Aero_CoorSys_V[Nm]/1(Out1) -> Mux1/2  "Trq_y_Aero_CoorSys_V[Nm]"
  Bus Selector5/5 -> Trq_y_Aero_CoorSys_V[Nm]/1(In1)  "<Trq_y_Aero_CoorSys_V[Nm]>"
  Trq_x_Aero_CoorSys_V[Nm]/1(Out1) -> Mux1/1  "Trq_x_Aero_CoorSys_V[Nm]"
  Bus Selector5/4 -> Trq_x_Aero_CoorSys_V[Nm]/1(In1)  "<Trq_x_Aero_CoorSys_V[Nm]>"
  F_z_Aero_CoorSys_V[N]/1(Out1) -> Mux/3  "F_z_Aero_CoorSys_V[N]"
  Bus Selector5/3 -> F_z_Aero_CoorSys_V[N]/1(In1)  "<F_z_Aero_CoorSys_V[N]>"
  F_y_Aero_CoorSys_V[N]/1(Out1) -> Mux/2  "F_y_Aero_CoorSys_V[N]"
  Bus Selector5/2 -> F_y_Aero_CoorSys_V[N]/1(In1)  "<F_y_Aero_CoorSys_V[N]>"
  F_x_Aero_CoorSys_V[N]/1(Out1) -> Mux/1  "F_x_Aero_CoorSys_V[N]"
  Bus Selector5/1 -> F_x_Aero_CoorSys_V[N]/1(In1)  "<F_x_Aero_CoorSys_V[N]>"
  Mux1/1 -> Aerodynamics1/2  "Trq_Aero[Nm]"
  Mux/1 -> Aerodynamics1/1  "F_Aero[N]"
  Aerodynamics/1 -> Bus Selector5/1

== system ASM_Traffic_V2X_Complete_Model_2/MDLUserInterface/VehicleDynamics/MDL_DISP/Brake ==
  Brake : Inport
  BrakeHydraulicsModel : Display
      settings: AttributesFormatString=1 - Complex\n2 - Basic
  BrakeHydraulicsModel[] : Subsystem
      mask Display: disp('')
  BrakePressure : Scope  NumInputPorts=6
  BrakeTorques : Scope  NumInputPorts=4
  Bus Selector2 : BusSelector  OutputSignals=BrakeHydraulics.BrakeHydraulicsModel[],BrakeDisc.Torque.Trq_FL_Brake[Nm],BrakeDisc.Torque.Trq_FR_Brake[Nm],BrakeDisc.Torque.Trq_RL_Brake[Nm],BrakeDisc.Torque.Trq_RR_Brake[Nm],MasterBrakeCylinder.ActiveBrakeCylinder.p[bar],MasterBrakeCylinder.ActiveBrakeCylinder.p_max[bar],BrakeDisc.Pressure.p_FL_Brake[bar],BrakeDisc.Pressure.p_FR_Brake[bar],BrakeDisc.Pressure.p_RL_Brake[bar],BrakeDisc.Pressure.p_RR_Brake[bar]
  Trq_FL_Brake[Nm] : Subsystem
      mask Display: disp('')
  Trq_FR_Brake[Nm] : Subsystem
      mask Display: disp('')
  Trq_RL_Brake[Nm] : Subsystem
      mask Display: disp('')
  Trq_RR_Brake[Nm] : Subsystem
      mask Display: disp('')
  p[bar] : Subsystem
      mask Display: disp('')
  p_FL_Brake[bar] : Subsystem
      mask Display: disp('')
  p_FR_Brake[bar] : Subsystem
      mask Display: disp('')
  p_RL_Brake[bar] : Subsystem
      mask Display: disp('')
  p_RR_Brake[bar] : Subsystem
      mask Display: disp('')
  p_max[bar] : Subsystem
      mask Display: disp('')
  wires:
  p_RR_Brake[bar]/1(Out1) -> BrakePressure/6  "p_RR_Brake[bar]"
  Bus Selector2/11 -> p_RR_Brake[bar]/1(In1)  "<p_RR_Brake[bar]>"
  p_RL_Brake[bar]/1(Out1) -> BrakePressure/5  "p_RL_Brake[bar]"
  Bus Selector2/10 -> p_RL_Brake[bar]/1(In1)  "<p_RL_Brake[bar]>"
  p_FR_Brake[bar]/1(Out1) -> BrakePressure/4  "p_FR_Brake[bar]"
  Bus Selector2/9 -> p_FR_Brake[bar]/1(In1)  "<p_FR_Brake[bar]>"
  p_FL_Brake[bar]/1(Out1) -> BrakePressure/3  "p_FL_Brake[bar]"
  Bus Selector2/8 -> p_FL_Brake[bar]/1(In1)  "<p_FL_Brake[bar]>"
  p_max[bar]/1(Out1) -> BrakePressure/2  "p_max[bar]"
  Bus Selector2/7 -> p_max[bar]/1(In1)  "<p_max[bar]>"
  p[bar]/1(Out1) -> BrakePressure/1  "p[bar]"
  Bus Selector2/6 -> p[bar]/1(In1)  "<p[bar]>"
  Trq_RR_Brake[Nm]/1(Out1) -> BrakeTorques/4  "Trq_RR_Brake[Nm]"
  Bus Selector2/5 -> Trq_RR_Brake[Nm]/1(In1)  "<Trq_RR_Brake[Nm]>"
  Trq_RL_Brake[Nm]/1(Out1) -> BrakeTorques/3  "Trq_RL_Brake[Nm]"
  Bus Selector2/4 -> Trq_RL_Brake[Nm]/1(In1)  "<Trq_RL_Brake[Nm]>"
  Trq_FR_Brake[Nm]/1(Out1) -> BrakeTorques/2  "Trq_FR_Brake[Nm]"
  Bus Selector2/3 -> Trq_FR_Brake[Nm]/1(In1)  "<Trq_FR_Brake[Nm]>"
  Trq_FL_Brake[Nm]/1(Out1) -> BrakeTorques/1  "Trq_FL_Brake[Nm]"
  Bus Selector2/2 -> Trq_FL_Brake[Nm]/1(In1)  "<Trq_FL_Brake[Nm]>"
  Brake/1 -> Bus Selector2/1
  BrakeHydraulicsModel[]/1(Out1) -> BrakeHydraulicsModel/1  "BrakeHydraulicsModel[]"
  Bus Selector2/1 -> BrakeHydraulicsModel[]/1(In1)  "<BrakeHydraulicsModel[]>"

== system ASM_Traffic_V2X_Complete_Model_2/MDLUserInterface/VehicleDynamics/MDL_DISP/Overview ==
  Velocities : Inport
  Accelerations : Inport  Port=2
  Bus Selector1 : BusSelector  OutputSignals=VehicleCoG.Linear.a_Vehicle_CoG[x;y;z][m|s2].a_x_Vehicle_CoG[m|s2],VehicleCoG.Linear.a_Vehicle_CoG[x;y;z][m|s2].a_y_Vehicle_CoG[m|s2],VehicleCoG.Linear.a_Vehicle_CoG[x;y;z][m|s2].a_z_Vehicle_CoG[m|s2]
  Bus Selector2 : BusSelector  OutputSignals=Vehicle.Linear.v_Vehicle_CoG[x;y;z][km|h].v_x_Vehicle_CoG[km|h],Vehicle.Linear.v_Vehicle_CoG[x;y;z][km|h].v_y_Vehicle_CoG[km|h],Vehicle.Linear.v_Vehicle_CoG[x;y;z][km|h].v_z_Vehicle_CoG[km|h],Vehicle.Linear.v_Total_Vehicle[km|h]
  Mux : Mux
  Mux1 : Mux  Inputs=3
  Overview : Scope  NumInputPorts=2
  a_x_Vehicle_CoG[m|s2] : Subsystem
      mask Display: disp('')
  a_y_Vehicle_CoG[m|s2] : Subsystem
      mask Display: disp('')
  a_z_Vehicle_CoG[m|s2] : Subsystem
      mask Display: disp('')
  v_Total_Vehicle[km|h] : Subsystem
      mask Display: disp('')
  v_x_Vehicle_CoG[km|h] : Subsystem
      mask Display: disp('')
  v_y_Vehicle_CoG[km|h] : Subsystem
      mask Display: disp('')
  v_z_Vehicle_CoG[km|h] : Subsystem
      mask Display: disp('')
  wires:
  Velocities/1 -> Bus Selector2/1
  Accelerations/1 -> Bus Selector1/1
  Mux/1 -> Overview/1  "Velocities"
  Mux1/1 -> Overview/2  "Accelerations"
  v_x_Vehicle_CoG[km|h]/1(Out1) -> Mux/1  "v_x_Vehicle_CoG[km|h]"
  v_y_Vehicle_CoG[km|h]/1(Out1) -> Mux/2  "v_y_Vehicle_CoG[km|h]"
  v_z_Vehicle_CoG[km|h]/1(Out1) -> Mux/3  "v_z_Vehicle_CoG[km|h]"
  v_Total_Vehicle[km|h]/1(Out1) -> Mux/4  "v_Total_Vehicle[km|h]"
  a_x_Vehicle_CoG[m|s2]/1(Out1) -> Mux1/1  "a_x_Vehicle_CoG[m|s2]"
  a_y_Vehicle_CoG[m|s2]/1(Out1) -> Mux1/2  "a_y_Vehicle_CoG[m|s2]"
  a_z_Vehicle_CoG[m|s2]/1(Out1) -> Mux1/3  "a_z_Vehicle_CoG[m|s2]"
  Bus Selector2/1 -> v_x_Vehicle_CoG[km|h]/1(In1)  "<v_x_Vehicle_CoG[km|h]>"
  Bus Selector2/2 -> v_y_Vehicle_CoG[km|h]/1(In1)  "<v_y_Vehicle_CoG[km|h]>"
  Bus Selector2/3 -> v_z_Vehicle_CoG[km|h]/1(In1)  "<v_z_Vehicle_CoG[km|h]>"
  Bus Selector2/4 -> v_Total_Vehicle[km|h]/1(In1)  "<v_Total_Vehicle[km|h]>"
  Bus Selector1/1 -> a_x_Vehicle_CoG[m|s2]/1(In1)  "<a_x_Vehicle_CoG[m|s2]>"
  Bus Selector1/2 -> a_y_Vehicle_CoG[m|s2]/1(In1)  "<a_y_Vehicle_CoG[m|s2]>"
  Bus Selector1/3 -> a_z_Vehicle_CoG[m|s2]/1(In1)  "<a_z_Vehicle_CoG[m|s2]>"

== system ASM_Traffic_V2X_Complete_Model_2/MDLUserInterface/VehicleDynamics/MDL_DISP/Positions ==
  Positions : Inport
  Angle_Pitch_Vehicle_CoorSys_E[deg] : Subsystem
      mask Display: disp('')
  Angle_Roll_Vehicle_CoorSys_E[deg] : Subsystem
      mask Display: disp('')
  Angle_Yaw_Vehicle_CoorSys_E[deg] : Subsystem
      mask Display: disp('')
  AngularPosition : Scope  NumInputPorts=3
  Bus Selector2 : BusSelector  OutputSignals=Vehicle.Linear.Pos_Vehicle_CoorSys_E[x;y;z][m].Pos_x_Vehicle_CoorSys_E[m],Vehicle.Linear.Pos_Vehicle_CoorSys_E[x;y;z][m].Pos_y_Vehicle_CoorSys_E[m],Vehicle.Linear.Pos_Vehicle_CoorSys_E[x;y;z][m].Pos_z_Vehicle_CoorSys_E[m],Vehicle.Linear.s_Vehicle[m],Vehicle.Angular.Angle_Vehicle_CoorSys_E[x;y;z][deg].Angle_Roll_Vehicle_CoorSys_E[deg],Vehicle.Angular.Angle_Vehicle_CoorSys_E[x;y;z][deg].Angle_Pitch_Vehicle_CoorSys_E[deg],Vehicle.Angular.Angle_Vehicle_CoorSys_E[x;y;z][deg].Angle_Yaw_Vehicle_CoorSys_E[deg]
  Pos_x_Vehicle_CoorSys_E[m] : Subsystem
      mask Display: disp('')
  Pos_y_Vehicle_CoorSys_E[m] : Subsystem
      mask Display: disp('')
  Pos_z_Vehicle_CoorSys_E[m] : Subsystem
      mask Display: disp('')
  TransPosition : Scope  NumInputPorts=4
  s_Vehicle[m] : Subsystem
      mask Display: disp('')
  wires:
  Positions/1 -> Bus Selector2/1
  Angle_Roll_Vehicle_CoorSys_E[deg]/1(Out1) -> AngularPosition/1  "Angle_Roll_Vehicle_CoorSys_E[deg]"
  Angle_Pitch_Vehicle_CoorSys_E[deg]/1(Out1) -> AngularPosition/2  "Angle_Pitch_Vehicle_CoorSys_E[deg]"
  Angle_Yaw_Vehicle_CoorSys_E[deg]/1(Out1) -> AngularPosition/3  "Angle_Yaw_Vehicle_CoorSys_E[deg]"
  Bus Selector2/5 -> Angle_Roll_Vehicle_CoorSys_E[deg]/1(In1)  "<Angle_Roll_Vehicle_CoorSys_E[deg]>"
  Bus Selector2/6 -> Angle_Pitch_Vehicle_CoorSys_E[deg]/1(In1)  "<Angle_Pitch_Vehicle_CoorSys_E[deg]>"
  Bus Selector2/7 -> Angle_Yaw_Vehicle_CoorSys_E[deg]/1(In1)  "<Angle_Yaw_Vehicle_CoorSys_E[deg]>"
  Pos_x_Vehicle_CoorSys_E[m]/1(Out1) -> TransPosition/1  "Pos_x_Vehicle_CoorSys_E[m]"
  Pos_y_Vehicle_CoorSys_E[m]/1(Out1) -> TransPosition/2  "Pos_y_Vehicle_CoorSys_E[m]"
  Pos_z_Vehicle_CoorSys_E[m]/1(Out1) -> TransPosition/3  "Pos_z_Vehicle_CoorSys_E[m]"
  s_Vehicle[m]/1(Out1) -> TransPosition/4  "s_Vehicle[m]"
  Bus Selector2/1 -> Pos_x_Vehicle_CoorSys_E[m]/1(In1)  "<Pos_x_Vehicle_CoorSys_E[m]>"
  Bus Selector2/2 -> Pos_y_Vehicle_CoorSys_E[m]/1(In1)  "<Pos_y_Vehicle_CoorSys_E[m]>"
  Bus Selector2/3 -> Pos_z_Vehicle_CoorSys_E[m]/1(In1)  "<Pos_z_Vehicle_CoorSys_E[m]>"
  Bus Selector2/4 -> s_Vehicle[m]/1(In1)  "<s_Vehicle[m]>"

== system ASM_Traffic_V2X_Complete_Model_2/MDLUserInterface/VehicleDynamics/MDL_DISP/Steering ==
  Steering : Inport
  Angle_SteeringGear[deg] : Subsystem
      mask Display: disp('')
  Angle_SteeringWheel[deg] : Subsystem
      mask Display: disp('')
  Bus Selector2 : BusSelector  OutputSignals=Displ_Steering[m],i_Steering_Mean[],ForcesAndTorques.TrqSpring_SteeringColumn[Nm],ForcesAndTorques.Trq_PowerSteering[Nm],Angle_SteeringWheel[deg],Angle_SteeringGear[deg]
  Displ_Steering[m] : Subsystem
      mask Display: disp('')
  SteeringSignals : Scope  NumInputPorts=6
  Trq_PowerSteering[Nm] : Subsystem
      mask Display: disp('')
  Trq_Steering[Nm] : Subsystem
      mask Display: disp('')
  i_Steering_Mean[] : Subsystem
      mask Display: disp('')
  wires:
  Steering/1 -> Bus Selector2/1
  Displ_Steering[m]/1(Out1) -> SteeringSignals/1  "Displ_Steering[m]"
  i_Steering_Mean[]/1(Out1) -> SteeringSignals/2  "i_Steering_Mean[]"
  Trq_Steering[Nm]/1(Out1) -> SteeringSignals/3  "Trq_Steering[Nm]"
  Trq_PowerSteering[Nm]/1(Out1) -> SteeringSignals/4  "Trq_PowerSteering[Nm]"
  Bus Selector2/1 -> Displ_Steering[m]/1(In1)  "<Displ_Steering[m]>"
  Bus Selector2/2 -> i_Steering_Mean[]/1(In1)  "<i_Steering_Mean[]>"
  Bus Selector2/3 -> Trq_Steering[Nm]/1(In1)  "<TrqSpring_SteeringColumn[Nm]>"
  Bus Selector2/4 -> Trq_PowerSteering[Nm]/1(In1)  "<Trq_PowerSteering[Nm]>"
  Bus Selector2/5 -> Angle_SteeringWheel[deg]/1(In1)  "<Angle_SteeringWheel[deg]>"
  Bus Selector2/6 -> Angle_SteeringGear[deg]/1(In1)  "<Angle_SteeringGear[deg]>"
  Angle_SteeringWheel[deg]/1(Out1) -> SteeringSignals/5  "Angle_SteeringWheel[deg]"
  Angle_SteeringGear[deg]/1(Out1) -> SteeringSignals/6  "Angle_SteeringGear[deg]"
